simulink model "ScriptDemo"  (R2022b)
settings: configuration reference "TmVcThermal_Configuration_sub" (kept outside this file)
undefined symbols (not defined in the file or in its folder): aaaa, bbbb, cTmComprCtrl_D_u8HvacFlowTable_db, cTmComprCtrl_D_u8HvacFlowTable_sw, cTmComprCtrl_n_i16ChillCmpIMax, cTmComprCtrl_n_i16ChillCmpIMin, cTmComprCtrl_n_i16ChillCmpIMin666, cTmComprCtrl_n_i16ChillCmpPMax, cTmComprCtrl_n_i16ChillCmpPMin, cTmComprCtrl_n_i16CmpChillCoolRpmKiMax, cTmComprCtrl_n_i16CmpChillCoolRpmKiMin, cTmComprCtrl_n_i16CmpChillCoolRpmKpMax, cTmComprCtrl_n_i16CmpChillCoolRpmKpMin, cTmComprCtrl_n_i16CmpCoolRpmKiMax, cTmComprCtrl_n_i16CmpCoolRpmKiMin, cTmComprCtrl_n_i16CmpCoolRpmKpMax, cTmComprCtrl_n_i16CmpCoolRpmKpMin, cTmComprCtrl_n_i16SM4CmpHeatKiMax, cTmComprCtrl_n_i16SM4CmpHeatKiMin, cTmComprCtrl_n_i16SM4CmpHeatKpMax, cTmComprCtrl_n_i16SM4CmpHeatKpMin, cTmComprCtrl_n_i16SM5CmpHeatKiMax, cTmComprCtrl_n_i16SM5CmpHeatKiMin, cTmComprCtrl_n_i16SM5CmpHeatKpMax, cTmComprCtrl_n_i16SM5CmpHeatKpMin, cTmComprCtrl_n_i16SM6CmpHeatKiMax, cTmComprCtrl_n_i16SM6CmpHeatKiMin, cTmComprCtrl_n_i16SM6CmpHeatKpMax, cTmComprCtrl_n_i16SM6CmpHeatKpMin, cTmComprCtrl_n_u16CmpMaxSpdFanFltLimt, cTmComprCtrl_n_u16CmpMaxSpdLoSidePFltLimt, cTmComprCtrl_n_u16CmpMaxSpdSensorFltLimt, cTmComprCtrl_n_u16CompMinRpm, cTmComprCtrl_n_u16CompRpmIncThres, cTmComprCtrl_t_u16BattCooltFFPeriod, cTmComprCtrl_t_u16BattCooltPIPeriod, cTmComprCtrl_t_u16CmpCoolFFPeriod, cTmComprCtrl_t_u16CmpCoolPIPeriod, cTmComprCtrl_t_u16CoolCmpChillFFPeriod, cTmComprCtrl_t_u16CoolCmpChillPIPeriod, cTmComprCtrl_t_u16SM4CmpHeatFFPeriod, cTmComprCtrl_t_u16SM4CmpHeatPIPeriod, cTmComprCtrl_t_u16SM5CmpHeatFFPeriod, cTmComprCtrl_t_u16SM5CmpHeatPIPeriod, cTmComprCtrl_t_u16SM6CmpHeatFFPeriod, cTmComprCtrl_t_u16SM6CmpHeatPIPeriod, cTmComprCtrl_Te_EvapClearInteg, cTmComprCtrl_Te_i16HpReqTempSaturoffset, cTmComprCtrl_Te_i16SatLpReplaceDiff, cTmComprCtrl_Te_i16SM3BatDiffStartEvapDecOffset, cTmComprCtrl_Te_i16SM3EvapLo, cTmComprCtrl_Te_i16SM3TBatDiffEntEvapDecOffset, cTmComprCtrl_Te_i16SM3TBatDiffEntEvapDecOffsetQuit, cTmComprCtrl_Te_s32ErrCmpChillPIContinueCoolH, cTmComprCtrl_Te_s32ErrCmpChillPIContinueCoolL, cTmComprCtrl_Te_s32ErrCmpPIContinueChillH, cTmComprCtrl_Te_s32ErrCmpPIContinueChillL, cTmComprCtrl_Te_s32ErrCmpPIContinueCoolH, cTmComprCtrl_Te_s32ErrCmpPIContinueCoolL, cTmComprCtrl_Te_s32ErrCmpPIContinueHeatH ... (+398)
libraries: simulink x846, PCMULib x711, simulink_need_slupdate x4
(part 23 of 49)

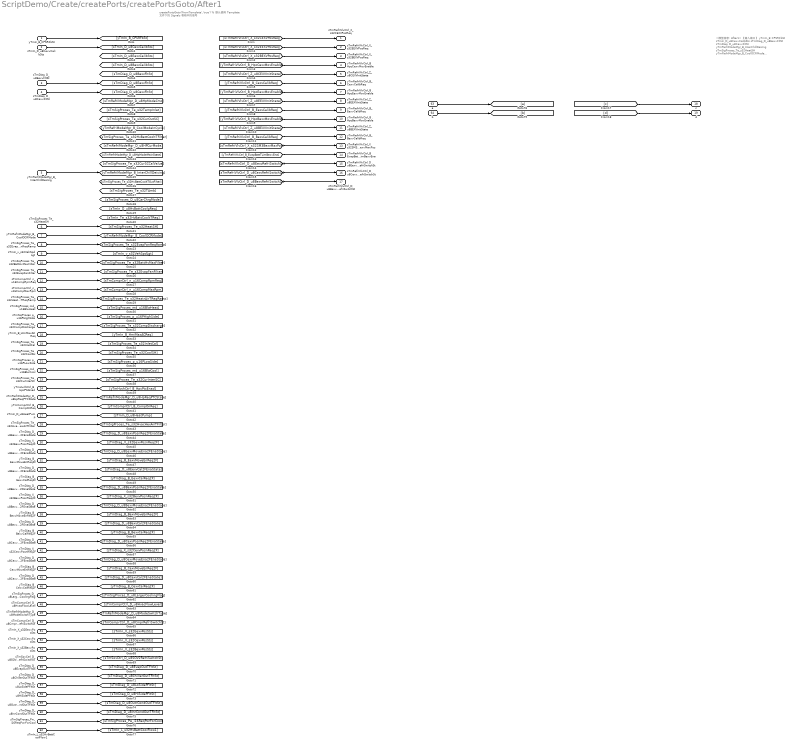
== system ScriptDemo/Create/createPorts/createPortsGoto/After1 ==
  note: createPortsGoto('fromTemplate','true')
      | % 默认使用 Template 文件下的 Signals 表格中的信号
  note: <模型信息: After1>
      |
      |
      | 【输入端口】
      | yTmIn_B_CPSRFbSt
      | sTmIn_D_u8CexvCalibSts
      | sTmDiag_D_u8EexvFltSt
      | sTmDiag_D_u8CexvFltSt
      | yTmRefriModeMgr_B_InterChillDeicing
      | sTmSigProces_Te_s32HeatSH
      | yTmRefriModeMgr_B_CoolOCRMode
      | sTmSigProces_Te_s32EvapFanReqRamp
      | sTmIn_v_s32VehSpdLgt
      | sTmSigProces_Te_s32BattHvMaxFilter
      | sTmSigProces_Te_s32EvapFanFilter
      | sTmComprCtrl_n_u16CompRpmReq
      | sTmComprCtrl_n_u16CompMaxRpm
      | sTmSigProces_Te_s32HeatrAirTReqRamp
      | sTmSigProces_md_u16BlwHeat
      | sTmSigProces_p_u16PHighSide
      | sTmSigProces_Te_s32CompDischarge
      | yTmIn_B_HmiMaxACReq
      | sTmSigProces_Te_s32InletCal
      | sTmSigProces_Te_s32CoolSH
      | sTmSigProces_p_u16PLowSide
      | sTmSigProces_md_u16BlwCool
      | sTmSigProces_Te_s32CurInterSC
      | yTmHvchCtrl_B_HpcPtcEnad
      | sTmRefriModeMgr_D_u8HpReqPTCState
      | yTmComprCtrl_B_CompOnReq
      | sTmIn_D_u8HeatPump
      | sTmSigProces_Te_s32HvacHexAirTFilter
      | sTmDiag_D_u8EexvPosnReq2FEnaState
      | sTmDiag_X_s32EexvPosnReq2F
      | sTmDiag_D_u8EexvMoveEna2FEnaState
      | yTmDiag_B_EexvMoveEnReq2F
      | sTmDiag_D_u8EexvCal2FEnaState
      | yTmDiag_B_EexvCalReq2F
      | sTmDiag_D_u8BexvPosnReq2FEnaState
      | sTmDiag_X_s32BexvPosnReq2F
      | sTmDiag_D_u8BexvMoveEna2FEnaState
      | yTmDiag_B_BexvMoveEnReq2F
      | sTmDiag_D_u8BexvCal2FEnaState
      | yTmDiag_B_BexvCalReq2F
      | sTmDiag_D_u8CexvPosnReq2FEnaState
      | sTmDiag_X_s32CexvPosnReq2F
      | sTmDiag_D_u8CexvMoveEna2FEnaState
      | yTmDiag_B_CexvMoveEnReq2F
      | sTmDiag_D_u8CexvCal2FEnaState
      | yTmDiag_B_CexvCalReq2F
      | sTmSigProces_D_u8LargerCoolingFlag
      | sTmComprCtrl_D_u8HvacFlowLevel
      | sTmRefriModeMgr_D_u8ModeSwitchType
      | sTmComprCtrl_D_u8CmprRefriSwitchSt
      | sTmIn_X_s32EexvPosSts
      | sTmIn_X_s32CexvPosSts
      | sTmIn_X_s32BexvPosSts
      | sTmSovCtrl_D_u8SOV2RefriSwitchSt
      | sTmDiag_D_u8EvapOutTFltSt
      | sTmDiag_D_u8ChillerOutTFltSt
      | sTmDiag_D_u8LoSidePFltSt
      | sTmDiag_D_u8HiSidePFltSt
      | sTmDiag_D_u8OutrCondOutTFltSt
      | sTmDiag_D_u8InrCondOutTFltSt
      | sTmSigProces_Pw_i16ReqPwrForCool
      | sTmIn_L_s32HvBattCoolFlow1
      | a
      | b
      |
      | 【输出端口】
      | sTmRefriVlvCtrl_X_s32CEXVPosReq
      | sTmRefriVlvCtrl_X_s32EEXVPosReq
      | sTmRefriVlvCtrl_X_s32BEXVPosReq
      | yTmRefriVlvCtrl_B_HpcCexvMovEnable
      | sTmRefriVlvCtrl_Z_u8CEXVInitState
      | yTmRefriVlvCtrl_B_CexvCalibReq
      | yTmRefriVlvCtrl_B_HpcEexvMovEnable
      | sTmRefriVlvCtrl_Z_u8EEXVInitState
      | yTmRefriVlvCtrl_B_EexvCalibReq
      | yTmRefriVlvCtrl_B_HpcBexvMovEnable
      | sTmRefriVlvCtrl_Z_u8BEXVInitState
      | yTmRefriVlvCtrl_B_BexvCalibReq
      | sTmRefriVlvCtrl_X_s32SM3BexvMaxPos
      | yTmRefriVlvCtrl_B_EvapBattTLimBexvEna
      | sTmRefriVlvCtrl_D_u8EexvRefriSwitchSt
      | sTmRefriVlvCtrl_D_u8CexvRefriSwitchSt
      | sTmRefriVlvCtrl_D_u8BexvRefriSwitchSt
      | c
      | d
      |
      | 【标定量】
      | 无标定量
      |
      | 创建时间: 2025-05-07 16:48:56
  yTmIn_B_CPSRFbSt : Inport  OutDataTypeStr=boolean
  sTmIn_D_u8CexvCalibSts : Inport  Port=2  OutDataTypeStr=uint8
  sTmDiag_D_u8EexvFltSt : Inport  Port=3  OutDataTypeStr=uint8
  sTmDiag_D_u8CexvFltSt : Inport  Port=4  OutDataTypeStr=uint8
  yTmRefriModeMgr_B_InterChillDeicing : Inport  Port=5  OutDataTypeStr=boolean
  sTmSigProces_Te_s32HeatSH : Inport  Port=6  OutDataTypeStr=single
  yTmRefriModeMgr_B_CoolOCRMode : Inport  Port=7  OutDataTypeStr=boolean
  sTmSigProces_Te_s32EvapFanReqRamp : Inport  Port=8  OutDataTypeStr=single
  sTmIn_v_s32VehSpdLgt : Inport  Port=9  OutDataTypeStr=single
  sTmSigProces_Te_s32BattHvMaxFilter : Inport  Port=10  OutDataTypeStr=single
  sTmSigProces_Te_s32EvapFanFilter : Inport  Port=11  OutDataTypeStr=single
  sTmComprCtrl_n_u16CompRpmReq : Inport  Port=12  OutDataTypeStr=uint16
  sTmComprCtrl_n_u16CompMaxRpm : Inport  Port=13  OutDataTypeStr=uint16
  sTmSigProces_Te_s32HeatrAirTReqRamp : Inport  Port=14  OutDataTypeStr=single
  sTmSigProces_md_u16BlwHeat : Inport  Port=15  OutDataTypeStr=uint16
  sTmSigProces_p_u16PHighSide : Inport  Port=16  OutDataTypeStr=uint16
  sTmSigProces_Te_s32CompDischarge : Inport  Port=17  OutDataTypeStr=single
  yTmIn_B_HmiMaxACReq : Inport  Port=18  OutDataTypeStr=boolean
  sTmSigProces_Te_s32InletCal : Inport  Port=19  OutDataTypeStr=single
  sTmSigProces_Te_s32CoolSH : Inport  Port=20  OutDataTypeStr=single
  sTmSigProces_p_u16PLowSide : Inport  Port=21  OutDataTypeStr=uint16
  sTmSigProces_md_u16BlwCool : Inport  Port=22  OutDataTypeStr=uint16
  sTmSigProces_Te_s32CurInterSC : Inport  Port=23  OutDataTypeStr=single
  yTmHvchCtrl_B_HpcPtcEnad : Inport  Port=24  OutDataTypeStr=boolean
  sTmRefriModeMgr_D_u8HpReqPTCState : Inport  Port=25  OutDataTypeStr=uint8
  yTmComprCtrl_B_CompOnReq : Inport  Port=26  OutDataTypeStr=boolean
  sTmIn_D_u8HeatPump : Inport  Port=27  OutDataTypeStr=uint8
  sTmSigProces_Te_s32HvacHexAirTFilter : Inport  Port=28  OutDataTypeStr=single
  sTmDiag_D_u8EexvPosnReq2FEnaState : Inport  Port=29  OutDataTypeStr=uint8
  sTmDiag_X_s32EexvPosnReq2F : Inport  Port=30  OutDataTypeStr=single
  sTmDiag_D_u8EexvMoveEna2FEnaState : Inport  Port=31  OutDataTypeStr=uint8
  yTmDiag_B_EexvMoveEnReq2F : Inport  Port=32  OutDataTypeStr=boolean
  sTmDiag_D_u8EexvCal2FEnaState : Inport  Port=33  OutDataTypeStr=uint8
  yTmDiag_B_EexvCalReq2F : Inport  Port=34  OutDataTypeStr=boolean
  sTmDiag_D_u8BexvPosnReq2FEnaState : Inport  Port=35  OutDataTypeStr=uint8
  sTmDiag_X_s32BexvPosnReq2F : Inport  Port=36  OutDataTypeStr=single
  sTmDiag_D_u8BexvMoveEna2FEnaState : Inport  Port=37  OutDataTypeStr=uint8
  yTmDiag_B_BexvMoveEnReq2F : Inport  Port=38  OutDataTypeStr=boolean
  sTmDiag_D_u8BexvCal2FEnaState : Inport  Port=39  OutDataTypeStr=uint8
  yTmDiag_B_BexvCalReq2F : Inport  Port=40  OutDataTypeStr=boolean
  sTmDiag_D_u8CexvPosnReq2FEnaState : Inport  Port=41  OutDataTypeStr=uint8
  sTmDiag_X_s32CexvPosnReq2F : Inport  Port=42  OutDataTypeStr=single
  sTmDiag_D_u8CexvMoveEna2FEnaState : Inport  Port=43  OutDataTypeStr=uint8
  yTmDiag_B_CexvMoveEnReq2F : Inport  Port=44  OutDataTypeStr=boolean
  sTmDiag_D_u8CexvCal2FEnaState : Inport  Port=45  OutDataTypeStr=uint8
  yTmDiag_B_CexvCalReq2F : Inport  Port=46  OutDataTypeStr=boolean
  sTmSigProces_D_u8LargerCoolingFlag : Inport  Port=47  OutDataTypeStr=uint8
  sTmComprCtrl_D_u8HvacFlowLevel : Inport  Port=48  OutDataTypeStr=uint8
  sTmRefriModeMgr_D_u8ModeSwitchType : Inport  Port=49  OutDataTypeStr=uint8
  sTmComprCtrl_D_u8CmprRefriSwitchSt : Inport  Port=50  OutDataTypeStr=uint8
  sTmIn_X_s32EexvPosSts : Inport  Port=51  OutDataTypeStr=single
  sTmIn_X_s32CexvPosSts : Inport  Port=52  OutDataTypeStr=single
  sTmIn_X_s32BexvPosSts : Inport  Port=53  OutDataTypeStr=single
  sTmSovCtrl_D_u8SOV2RefriSwitchSt : Inport  Port=54  OutDataTypeStr=uint8
  sTmDiag_D_u8EvapOutTFltSt : Inport  Port=55  OutDataTypeStr=uint8
  sTmDiag_D_u8ChillerOutTFltSt : Inport  Port=56  OutDataTypeStr=uint8
  sTmDiag_D_u8LoSidePFltSt : Inport  Port=57  OutDataTypeStr=uint8
  sTmDiag_D_u8HiSidePFltSt : Inport  Port=58  OutDataTypeStr=uint8
  sTmDiag_D_u8OutrCondOutTFltSt : Inport  Port=59  OutDataTypeStr=uint8
  sTmDiag_D_u8InrCondOutTFltSt : Inport  Port=60  OutDataTypeStr=uint8
  sTmSigProces_Pw_i16ReqPwrForCool : Inport  Port=61  OutDataTypeStr=int16
  sTmIn_L_s32HvBattCoolFlow1 : Inport  Port=62  OutDataTypeStr=single
  a : Inport  Port=63
  b : Inport  Port=64
  sTmRefriVlvCtrl_X_s32CEXVPosReq : Outport  OutDataTypeStr=single
  sTmRefriVlvCtrl_X_s32EEXVPosReq : Outport  Port=2  OutDataTypeStr=single
  sTmRefriVlvCtrl_X_s32BEXVPosReq : Outport  Port=3  OutDataTypeStr=single
  yTmRefriVlvCtrl_B_HpcCexvMovEnable : Outport  Port=4  OutDataTypeStr=boolean
  sTmRefriVlvCtrl_Z_u8CEXVInitState : Outport  Port=5  OutDataTypeStr=uint8
  yTmRefriVlvCtrl_B_CexvCalibReq : Outport  Port=6  OutDataTypeStr=boolean
  yTmRefriVlvCtrl_B_HpcEexvMovEnable : Outport  Port=7  OutDataTypeStr=boolean
  sTmRefriVlvCtrl_Z_u8EEXVInitState : Outport  Port=8  OutDataTypeStr=uint8
  yTmRefriVlvCtrl_B_EexvCalibReq : Outport  Port=9  OutDataTypeStr=boolean
  yTmRefriVlvCtrl_B_HpcBexvMovEnable : Outport  Port=10  OutDataTypeStr=boolean
  sTmRefriVlvCtrl_Z_u8BEXVInitState : Outport  Port=11  OutDataTypeStr=uint8
  yTmRefriVlvCtrl_B_BexvCalibReq : Outport  Port=12  OutDataTypeStr=boolean
  sTmRefriVlvCtrl_X_s32SM3BexvMaxPos : Outport  Port=13  OutDataTypeStr=single
  yTmRefriVlvCtrl_B_EvapBattTLimBexvEna : Outport  Port=14  OutDataTypeStr=boolean
  sTmRefriVlvCtrl_D_u8EexvRefriSwitchSt : Outport  Port=15  OutDataTypeStr=uint8
  sTmRefriVlvCtrl_D_u8CexvRefriSwitchSt : Outport  Port=16  OutDataTypeStr=uint8
  sTmRefriVlvCtrl_D_u8BexvRefriSwitchSt : Outport  Port=17  OutDataTypeStr=uint8
  c : Outport  Port=18
  d : Outport  Port=19
  wires:
  yTmIn_B_CPSRFbSt/1 -> [yTmIn_B_CPSRFbSt]
  sTmIn_D_u8CexvCalibSts/1 -> [sTmIn_D_u8CexvCalibSts]
  ? -> [sTmIn_D_u8EexvCalibSts]
  ? -> [sTmIn_D_u8BexvCalibSts]
  ? -> [sTmDiag_D_u8BexvFltSt]
  sTmDiag_D_u8EexvFltSt/1 -> [sTmDiag_D_u8EexvFltSt]
  sTmDiag_D_u8CexvFltSt/1 -> [sTmDiag_D_u8CexvFltSt]
  ? -> [sTmRefriModeMgr_D_u8HpModeCmd]
  ? -> [sTmSigProces_Te_s32TempInlet]
  ? -> [sTmSigProces_Te_s32CurOutSC]
  ? -> [yTmRefriModeMgr_B_CoolModeInCycle]
  ? -> [sTmSigProces_Te_s32HvBattCooltTFilter]
  ? -> [sTmRefriModeMgr_D_u8HPCurMode]
  ? -> [sTmRefriModeMgr_D_u8HpModeMainState]
  ? -> [sTmSigProces_Te_s32CurSCCalValue]
  yTmRefriModeMgr_B_InterChillDeicing/1 -> [yTmRefriModeMgr_B_InterChillDeicing]
  ? -> [sTmSigProces_Te_s32HvBattCooltTOutFilter]
  ? -> [sTmSigProces_Te_s32TAmb]
  ? -> [sTmSigProces_D_u8CarChrgMode]
  ? -> [sTmIn_D_u8HvBattCoolgReq]
  ? -> [sTmIn_Te_s32HvBattCooltTReq]
  sTmSigProces_Te_s32HeatSH/1 -> [sTmSigProces_Te_s32HeatSH]
  yTmRefriModeMgr_B_CoolOCRMode/1 -> [yTmRefriModeMgr_B_CoolOCRMode]
  sTmSigProces_Te_s32EvapFanReqRamp/1 -> [sTmSigProces_Te_s32EvapFanReqRamp]
  sTmIn_v_s32VehSpdLgt/1 -> [sTmIn_v_s32VehSpdLgt]
  sTmSigProces_Te_s32BattHvMaxFilter/1 -> [sTmSigProces_Te_s32BattHvMaxFilter]
  sTmSigProces_Te_s32EvapFanFilter/1 -> [sTmSigProces_Te_s32EvapFanFilter]
  sTmComprCtrl_n_u16CompRpmReq/1 -> [sTmComprCtrl_n_u16CompRpmReq]
  sTmComprCtrl_n_u16CompMaxRpm/1 -> [sTmComprCtrl_n_u16CompMaxRpm]
  sTmSigProces_Te_s32HeatrAirTReqRamp/1 -> [sTmSigProces_Te_s32HeatrAirTReqRamp]
  sTmSigProces_md_u16BlwHeat/1 -> [sTmSigProces_md_u16BlwHeat]
  sTmSigProces_p_u16PHighSide/1 -> [sTmSigProces_p_u16PHighSide]
  sTmSigProces_Te_s32CompDischarge/1 -> [sTmSigProces_Te_s32CompDischarge]
  yTmIn_B_HmiMaxACReq/1 -> [yTmIn_B_HmiMaxACReq]
  sTmSigProces_Te_s32InletCal/1 -> [sTmSigProces_Te_s32InletCal]
  sTmSigProces_Te_s32CoolSH/1 -> [sTmSigProces_Te_s32CoolSH]
  sTmSigProces_p_u16PLowSide/1 -> [sTmSigProces_p_u16PLowSide]
  sTmSigProces_md_u16BlwCool/1 -> [sTmSigProces_md_u16BlwCool]
  sTmSigProces_Te_s32CurInterSC/1 -> [sTmSigProces_Te_s32CurInterSC]
  yTmHvchCtrl_B_HpcPtcEnad/1 -> [yTmHvchCtrl_B_HpcPtcEnad]
  sTmRefriModeMgr_D_u8HpReqPTCState/1 -> [sTmRefriModeMgr_D_u8HpReqPTCState]
  yTmComprCtrl_B_CompOnReq/1 -> [yTmComprCtrl_B_CompOnReq]
  sTmIn_D_u8HeatPump/1 -> [sTmIn_D_u8HeatPump]
  sTmSigProces_Te_s32HvacHexAirTFilter/1 -> [sTmSigProces_Te_s32HvacHexAirTFilter]
  sTmDiag_D_u8EexvPosnReq2FEnaState/1 -> [sTmDiag_D_u8EexvPosnReq2FEnaState]
  sTmDiag_X_s32EexvPosnReq2F/1 -> [sTmDiag_X_s32EexvPosnReq2F]
  sTmDiag_D_u8EexvMoveEna2FEnaState/1 -> [sTmDiag_D_u8EexvMoveEna2FEnaState]
  yTmDiag_B_EexvMoveEnReq2F/1 -> [yTmDiag_B_EexvMoveEnReq2F]
  sTmDiag_D_u8EexvCal2FEnaState/1 -> [sTmDiag_D_u8EexvCal2FEnaState]
  yTmDiag_B_EexvCalReq2F/1 -> [yTmDiag_B_EexvCalReq2F]
  sTmDiag_D_u8BexvPosnReq2FEnaState/1 -> [sTmDiag_D_u8BexvPosnReq2FEnaState]
  sTmDiag_X_s32BexvPosnReq2F/1 -> [sTmDiag_X_s32BexvPosnReq2F]
  sTmDiag_D_u8BexvMoveEna2FEnaState/1 -> [sTmDiag_D_u8BexvMoveEna2FEnaState]
  yTmDiag_B_BexvMoveEnReq2F/1 -> [yTmDiag_B_BexvMoveEnReq2F]
  sTmDiag_D_u8BexvCal2FEnaState/1 -> [sTmDiag_D_u8BexvCal2FEnaState]
  yTmDiag_B_BexvCalReq2F/1 -> [yTmDiag_B_BexvCalReq2F]
  sTmDiag_D_u8CexvPosnReq2FEnaState/1 -> [sTmDiag_D_u8CexvPosnReq2FEnaState]
  sTmDiag_X_s32CexvPosnReq2F/1 -> [sTmDiag_X_s32CexvPosnReq2F]
  sTmDiag_D_u8CexvMoveEna2FEnaState/1 -> [sTmDiag_D_u8CexvMoveEna2FEnaState]
  yTmDiag_B_CexvMoveEnReq2F/1 -> [yTmDiag_B_CexvMoveEnReq2F]
  sTmDiag_D_u8CexvCal2FEnaState/1 -> [sTmDiag_D_u8CexvCal2FEnaState]
  yTmDiag_B_CexvCalReq2F/1 -> [yTmDiag_B_CexvCalReq2F]
  sTmSigProces_D_u8LargerCoolingFlag/1 -> [sTmSigProces_D_u8LargerCoolingFlag]
  sTmComprCtrl_D_u8HvacFlowLevel/1 -> [sTmComprCtrl_D_u8HvacFlowLevel]
  sTmRefriModeMgr_D_u8ModeSwitchType/1 -> [sTmRefriModeMgr_D_u8ModeSwitchType]
  sTmComprCtrl_D_u8CmprRefriSwitchSt/1 -> [sTmComprCtrl_D_u8CmprRefriSwitchSt]
  sTmIn_X_s32EexvPosSts/1 -> [sTmIn_X_s32EexvPosSts]
  sTmIn_X_s32CexvPosSts/1 -> [sTmIn_X_s32CexvPosSts]
  sTmIn_X_s32BexvPosSts/1 -> [sTmIn_X_s32BexvPosSts]
  sTmSovCtrl_D_u8SOV2RefriSwitchSt/1 -> [sTmSovCtrl_D_u8SOV2RefriSwitchSt]
  sTmDiag_D_u8EvapOutTFltSt/1 -> [sTmDiag_D_u8EvapOutTFltSt]
  sTmDiag_D_u8ChillerOutTFltSt/1 -> [sTmDiag_D_u8ChillerOutTFltSt]
  sTmDiag_D_u8LoSidePFltSt/1 -> [sTmDiag_D_u8LoSidePFltSt]
  sTmDiag_D_u8HiSidePFltSt/1 -> [sTmDiag_D_u8HiSidePFltSt]
  sTmDiag_D_u8OutrCondOutTFltSt/1 -> [sTmDiag_D_u8OutrCondOutTFltSt]
  sTmDiag_D_u8InrCondOutTFltSt/1 -> [sTmDiag_D_u8InrCondOutTFltSt]
  sTmSigProces_Pw_i16ReqPwrForCool/1 -> [sTmSigProces_Pw_i16ReqPwrForCool]
  sTmIn_L_s32HvBattCoolFlow1/1 -> [sTmIn_L_s32HvBattCoolFlow1]
  [sTmRefriVlvCtrl_X_s32CEXVPosReq] -> sTmRefriVlvCtrl_X_s32CEXVPosReq/1
  [sTmRefriVlvCtrl_X_s32EEXVPosReq] -> sTmRefriVlvCtrl_X_s32EEXVPosReq/1
  [sTmRefriVlvCtrl_X_s32BEXVPosReq] -> sTmRefriVlvCtrl_X_s32BEXVPosReq/1
  [yTmRefriVlvCtrl_B_HpcCexvMovEnable] -> yTmRefriVlvCtrl_B_HpcCexvMovEnable/1
  [sTmRefriVlvCtrl_Z_u8CEXVInitState] -> sTmRefriVlvCtrl_Z_u8CEXVInitState/1
  [yTmRefriVlvCtrl_B_CexvCalibReq] -> yTmRefriVlvCtrl_B_CexvCalibReq/1
  [yTmRefriVlvCtrl_B_HpcEexvMovEnable] -> yTmRefriVlvCtrl_B_HpcEexvMovEnable/1
  [sTmRefriVlvCtrl_Z_u8EEXVInitState] -> sTmRefriVlvCtrl_Z_u8EEXVInitState/1
  [yTmRefriVlvCtrl_B_EexvCalibReq] -> yTmRefriVlvCtrl_B_EexvCalibReq/1
  [yTmRefriVlvCtrl_B_HpcBexvMovEnable] -> yTmRefriVlvCtrl_B_HpcBexvMovEnable/1
  [sTmRefriVlvCtrl_Z_u8BEXVInitState] -> sTmRefriVlvCtrl_Z_u8BEXVInitState/1
  [yTmRefriVlvCtrl_B_BexvCalibReq] -> yTmRefriVlvCtrl_B_BexvCalibReq/1
  [sTmRefriVlvCtrl_X_s32SM3BexvMaxPos] -> sTmRefriVlvCtrl_X_s32SM3BexvMaxPos/1
  [yTmRefriVlvCtrl_B_EvapBattTLimBexvEna] -> yTmRefriVlvCtrl_B_EvapBattTLimBexvEna/1
  [sTmRefriVlvCtrl_D_u8EexvRefriSwitchSt] -> sTmRefriVlvCtrl_D_u8EexvRefriSwitchSt/1
  [sTmRefriVlvCtrl_D_u8CexvRefriSwitchSt] -> sTmRefriVlvCtrl_D_u8CexvRefriSwitchSt/1
  [sTmRefriVlvCtrl_D_u8BexvRefriSwitchSt] -> sTmRefriVlvCtrl_D_u8BexvRefriSwitchSt/1
  a/1 -> [a]
  b/1 -> [b]
  [c] -> c/1
  [d] -> d/1

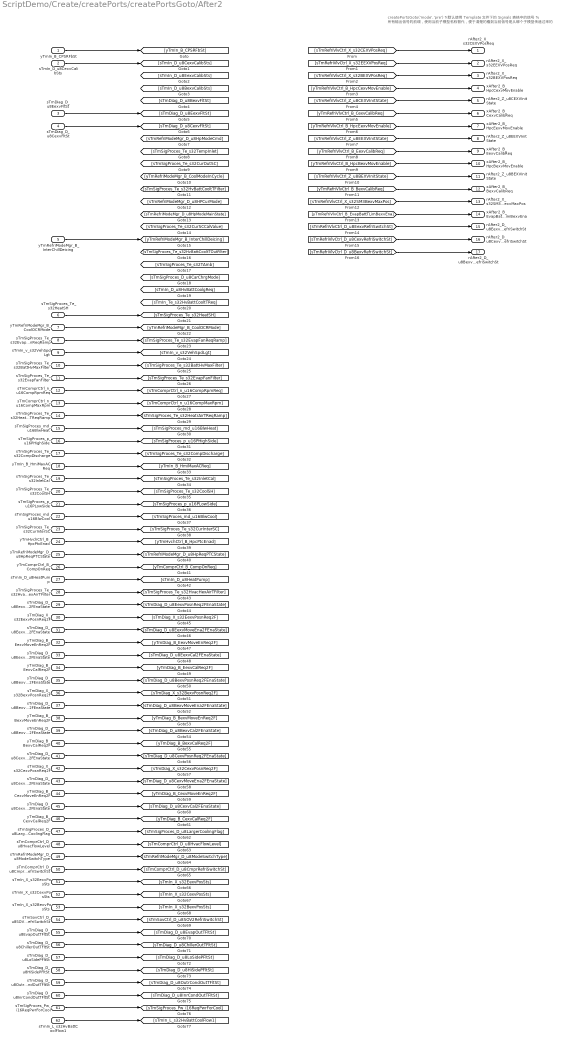
== system ScriptDemo/Create/createPorts/createPortsGoto/After2 ==
  note: createPortsGoto('mode','pre')
      | % 默认使用 Template 文件下的 Signals 表格中的信号
      | % 所有输出信号的前缀，使用当前子模型名称替代，便于清楚的看到当前信号是从哪个子模型传递过来的
  yTmIn_B_CPSRFbSt : Inport  OutDataTypeStr=boolean
  sTmIn_D_u8CexvCalibSts : Inport  Port=2  OutDataTypeStr=uint8
  sTmDiag_D_u8EexvFltSt : Inport  Port=3  OutDataTypeStr=uint8
  sTmDiag_D_u8CexvFltSt : Inport  Port=4  OutDataTypeStr=uint8
  yTmRefriModeMgr_B_InterChillDeicing : Inport  Port=5  OutDataTypeStr=boolean
  sTmSigProces_Te_s32HeatSH : Inport  Port=6  OutDataTypeStr=single
  yTmRefriModeMgr_B_CoolOCRMode : Inport  Port=7  OutDataTypeStr=boolean
  sTmSigProces_Te_s32EvapFanReqRamp : Inport  Port=8  OutDataTypeStr=single
  sTmIn_v_s32VehSpdLgt : Inport  Port=9  OutDataTypeStr=single
  sTmSigProces_Te_s32BattHvMaxFilter : Inport  Port=10  OutDataTypeStr=single
  sTmSigProces_Te_s32EvapFanFilter : Inport  Port=11  OutDataTypeStr=single
  sTmComprCtrl_n_u16CompRpmReq : Inport  Port=12  OutDataTypeStr=uint16
  sTmComprCtrl_n_u16CompMaxRpm : Inport  Port=13  OutDataTypeStr=uint16
  sTmSigProces_Te_s32HeatrAirTReqRamp : Inport  Port=14  OutDataTypeStr=single
  sTmSigProces_md_u16BlwHeat : Inport  Port=15  OutDataTypeStr=uint16
  sTmSigProces_p_u16PHighSide : Inport  Port=16  OutDataTypeStr=uint16
  sTmSigProces_Te_s32CompDischarge : Inport  Port=17  OutDataTypeStr=single
  yTmIn_B_HmiMaxACReq : Inport  Port=18  OutDataTypeStr=boolean
  sTmSigProces_Te_s32InletCal : Inport  Port=19  OutDataTypeStr=single
  sTmSigProces_Te_s32CoolSH : Inport  Port=20  OutDataTypeStr=single
  sTmSigProces_p_u16PLowSide : Inport  Port=21  OutDataTypeStr=uint16
  sTmSigProces_md_u16BlwCool : Inport  Port=22  OutDataTypeStr=uint16
  sTmSigProces_Te_s32CurInterSC : Inport  Port=23  OutDataTypeStr=single
  yTmHvchCtrl_B_HpcPtcEnad : Inport  Port=24  OutDataTypeStr=boolean
  sTmRefriModeMgr_D_u8HpReqPTCState : Inport  Port=25  OutDataTypeStr=uint8
  yTmComprCtrl_B_CompOnReq : Inport  Port=26  OutDataTypeStr=boolean
  sTmIn_D_u8HeatPump : Inport  Port=27  OutDataTypeStr=uint8
  sTmSigProces_Te_s32HvacHexAirTFilter : Inport  Port=28  OutDataTypeStr=single
  sTmDiag_D_u8EexvPosnReq2FEnaState : Inport  Port=29  OutDataTypeStr=uint8
  sTmDiag_X_s32EexvPosnReq2F : Inport  Port=30  OutDataTypeStr=single
  sTmDiag_D_u8EexvMoveEna2FEnaState : Inport  Port=31  OutDataTypeStr=uint8
  yTmDiag_B_EexvMoveEnReq2F : Inport  Port=32  OutDataTypeStr=boolean
  sTmDiag_D_u8EexvCal2FEnaState : Inport  Port=33  OutDataTypeStr=uint8
  yTmDiag_B_EexvCalReq2F : Inport  Port=34  OutDataTypeStr=boolean
  sTmDiag_D_u8BexvPosnReq2FEnaState : Inport  Port=35  OutDataTypeStr=uint8
  sTmDiag_X_s32BexvPosnReq2F : Inport  Port=36  OutDataTypeStr=single
  sTmDiag_D_u8BexvMoveEna2FEnaState : Inport  Port=37  OutDataTypeStr=uint8
  yTmDiag_B_BexvMoveEnReq2F : Inport  Port=38  OutDataTypeStr=boolean
  sTmDiag_D_u8BexvCal2FEnaState : Inport  Port=39  OutDataTypeStr=uint8
  yTmDiag_B_BexvCalReq2F : Inport  Port=40  OutDataTypeStr=boolean
  sTmDiag_D_u8CexvPosnReq2FEnaState : Inport  Port=41  OutDataTypeStr=uint8
  sTmDiag_X_s32CexvPosnReq2F : Inport  Port=42  OutDataTypeStr=single
  sTmDiag_D_u8CexvMoveEna2FEnaState : Inport  Port=43  OutDataTypeStr=uint8
  yTmDiag_B_CexvMoveEnReq2F : Inport  Port=44  OutDataTypeStr=boolean
  sTmDiag_D_u8CexvCal2FEnaState : Inport  Port=45  OutDataTypeStr=uint8
  yTmDiag_B_CexvCalReq2F : Inport  Port=46  OutDataTypeStr=boolean
  sTmSigProces_D_u8LargerCoolingFlag : Inport  Port=47  OutDataTypeStr=uint8
  sTmComprCtrl_D_u8HvacFlowLevel : Inport  Port=48  OutDataTypeStr=uint8
  sTmRefriModeMgr_D_u8ModeSwitchType : Inport  Port=49  OutDataTypeStr=uint8
  sTmComprCtrl_D_u8CmprRefriSwitchSt : Inport  Port=50  OutDataTypeStr=uint8
  sTmIn_X_s32EexvPosSts : Inport  Port=51  OutDataTypeStr=single
  sTmIn_X_s32CexvPosSts : Inport  Port=52  OutDataTypeStr=single
  sTmIn_X_s32BexvPosSts : Inport  Port=53  OutDataTypeStr=single
  sTmSovCtrl_D_u8SOV2RefriSwitchSt : Inport  Port=54  OutDataTypeStr=uint8
  sTmDiag_D_u8EvapOutTFltSt : Inport  Port=55  OutDataTypeStr=uint8
  sTmDiag_D_u8ChillerOutTFltSt : Inport  Port=56  OutDataTypeStr=uint8
  sTmDiag_D_u8LoSidePFltSt : Inport  Port=57  OutDataTypeStr=uint8
  sTmDiag_D_u8HiSidePFltSt : Inport  Port=58  OutDataTypeStr=uint8
  sTmDiag_D_u8OutrCondOutTFltSt : Inport  Port=59  OutDataTypeStr=uint8
  sTmDiag_D_u8InrCondOutTFltSt : Inport  Port=60  OutDataTypeStr=uint8
  sTmSigProces_Pw_i16ReqPwrForCool : Inport  Port=61  OutDataTypeStr=int16
  sTmIn_L_s32HvBattCoolFlow1 : Inport  Port=62  OutDataTypeStr=single
  rAfter2_X_s32CEXVPosReq : Outport  OutDataTypeStr=single
  rAfter2_X_s32EEXVPosReq : Outport  Port=2  OutDataTypeStr=single
  rAfter2_X_s32BEXVPosReq : Outport  Port=3  OutDataTypeStr=single
  xAfter2_B_HpcCexvMovEnable : Outport  Port=4  OutDataTypeStr=boolean
  rAfter2_Z_u8CEXVInitState : Outport  Port=5  OutDataTypeStr=uint8
  xAfter2_B_CexvCalibReq : Outport  Port=6  OutDataTypeStr=boolean
  xAfter2_B_HpcEexvMovEnable : Outport  Port=7  OutDataTypeStr=boolean
  rAfter2_Z_u8EEXVInitState : Outport  Port=8  OutDataTypeStr=uint8
  xAfter2_B_EexvCalibReq : Outport  Port=9  OutDataTypeStr=boolean
  xAfter2_B_HpcBexvMovEnable : Outport  Port=10  OutDataTypeStr=boolean
  rAfter2_Z_u8BEXVInitState : Outport  Port=11  OutDataTypeStr=uint8
  xAfter2_B_BexvCalibReq : Outport  Port=12  OutDataTypeStr=boolean
  rAfter2_X_s32SM3BexvMaxPos : Outport  Port=13  OutDataTypeStr=single
  xAfter2_B_EvapBattTLimBexvEna : Outport  Port=14  OutDataTypeStr=boolean
  rAfter2_D_u8EexvRefriSwitchSt : Outport  Port=15  OutDataTypeStr=uint8
  rAfter2_D_u8CexvRefriSwitchSt : Outport  Port=16  OutDataTypeStr=uint8
  rAfter2_D_u8BexvRefriSwitchSt : Outport  Port=17  OutDataTypeStr=uint8
  wires:
  yTmIn_B_CPSRFbSt/1 -> [yTmIn_B_CPSRFbSt]
  sTmIn_D_u8CexvCalibSts/1 -> [sTmIn_D_u8CexvCalibSts]
  ? -> [sTmIn_D_u8EexvCalibSts]
  ? -> [sTmIn_D_u8BexvCalibSts]
  ? -> [sTmDiag_D_u8BexvFltSt]
  sTmDiag_D_u8EexvFltSt/1 -> [sTmDiag_D_u8EexvFltSt]
  sTmDiag_D_u8CexvFltSt/1 -> [sTmDiag_D_u8CexvFltSt]
  ? -> [sTmRefriModeMgr_D_u8HpModeCmd]
  ? -> [sTmSigProces_Te_s32TempInlet]
  ? -> [sTmSigProces_Te_s32CurOutSC]
  ? -> [yTmRefriModeMgr_B_CoolModeInCycle]
  ? -> [sTmSigProces_Te_s32HvBattCooltTFilter]
  ? -> [sTmRefriModeMgr_D_u8HPCurMode]
  ? -> [sTmRefriModeMgr_D_u8HpModeMainState]
  ? -> [sTmSigProces_Te_s32CurSCCalValue]
  yTmRefriModeMgr_B_InterChillDeicing/1 -> [yTmRefriModeMgr_B_InterChillDeicing]
  ? -> [sTmSigProces_Te_s32HvBattCooltTOutFilter]
  ? -> [sTmSigProces_Te_s32TAmb]
  ? -> [sTmSigProces_D_u8CarChrgMode]
  ? -> [sTmIn_D_u8HvBattCoolgReq]
  ? -> [sTmIn_Te_s32HvBattCooltTReq]
  sTmSigProces_Te_s32HeatSH/1 -> [sTmSigProces_Te_s32HeatSH]
  yTmRefriModeMgr_B_CoolOCRMode/1 -> [yTmRefriModeMgr_B_CoolOCRMode]
  sTmSigProces_Te_s32EvapFanReqRamp/1 -> [sTmSigProces_Te_s32EvapFanReqRamp]
  sTmIn_v_s32VehSpdLgt/1 -> [sTmIn_v_s32VehSpdLgt]
  sTmSigProces_Te_s32BattHvMaxFilter/1 -> [sTmSigProces_Te_s32BattHvMaxFilter]
  sTmSigProces_Te_s32EvapFanFilter/1 -> [sTmSigProces_Te_s32EvapFanFilter]
  sTmComprCtrl_n_u16CompRpmReq/1 -> [sTmComprCtrl_n_u16CompRpmReq]
  sTmComprCtrl_n_u16CompMaxRpm/1 -> [sTmComprCtrl_n_u16CompMaxRpm]
  sTmSigProces_Te_s32HeatrAirTReqRamp/1 -> [sTmSigProces_Te_s32HeatrAirTReqRamp]
  sTmSigProces_md_u16BlwHeat/1 -> [sTmSigProces_md_u16BlwHeat]
  sTmSigProces_p_u16PHighSide/1 -> [sTmSigProces_p_u16PHighSide]
  sTmSigProces_Te_s32CompDischarge/1 -> [sTmSigProces_Te_s32CompDischarge]
  yTmIn_B_HmiMaxACReq/1 -> [yTmIn_B_HmiMaxACReq]
  sTmSigProces_Te_s32InletCal/1 -> [sTmSigProces_Te_s32InletCal]
  sTmSigProces_Te_s32CoolSH/1 -> [sTmSigProces_Te_s32CoolSH]
  sTmSigProces_p_u16PLowSide/1 -> [sTmSigProces_p_u16PLowSide]
  sTmSigProces_md_u16BlwCool/1 -> [sTmSigProces_md_u16BlwCool]
  sTmSigProces_Te_s32CurInterSC/1 -> [sTmSigProces_Te_s32CurInterSC]
  yTmHvchCtrl_B_HpcPtcEnad/1 -> [yTmHvchCtrl_B_HpcPtcEnad]
  sTmRefriModeMgr_D_u8HpReqPTCState/1 -> [sTmRefriModeMgr_D_u8HpReqPTCState]
  yTmComprCtrl_B_CompOnReq/1 -> [yTmComprCtrl_B_CompOnReq]
  sTmIn_D_u8HeatPump/1 -> [sTmIn_D_u8HeatPump]
  sTmSigProces_Te_s32HvacHexAirTFilter/1 -> [sTmSigProces_Te_s32HvacHexAirTFilter]
  sTmDiag_D_u8EexvPosnReq2FEnaState/1 -> [sTmDiag_D_u8EexvPosnReq2FEnaState]
  sTmDiag_X_s32EexvPosnReq2F/1 -> [sTmDiag_X_s32EexvPosnReq2F]
  sTmDiag_D_u8EexvMoveEna2FEnaState/1 -> [sTmDiag_D_u8EexvMoveEna2FEnaState]
  yTmDiag_B_EexvMoveEnReq2F/1 -> [yTmDiag_B_EexvMoveEnReq2F]
  sTmDiag_D_u8EexvCal2FEnaState/1 -> [sTmDiag_D_u8EexvCal2FEnaState]
  yTmDiag_B_EexvCalReq2F/1 -> [yTmDiag_B_EexvCalReq2F]
  sTmDiag_D_u8BexvPosnReq2FEnaState/1 -> [sTmDiag_D_u8BexvPosnReq2FEnaState]
  sTmDiag_X_s32BexvPosnReq2F/1 -> [sTmDiag_X_s32BexvPosnReq2F]
  sTmDiag_D_u8BexvMoveEna2FEnaState/1 -> [sTmDiag_D_u8BexvMoveEna2FEnaState]
  yTmDiag_B_BexvMoveEnReq2F/1 -> [yTmDiag_B_BexvMoveEnReq2F]
  sTmDiag_D_u8BexvCal2FEnaState/1 -> [sTmDiag_D_u8BexvCal2FEnaState]
  yTmDiag_B_BexvCalReq2F/1 -> [yTmDiag_B_BexvCalReq2F]
  sTmDiag_D_u8CexvPosnReq2FEnaState/1 -> [sTmDiag_D_u8CexvPosnReq2FEnaState]
  sTmDiag_X_s32CexvPosnReq2F/1 -> [sTmDiag_X_s32CexvPosnReq2F]
  sTmDiag_D_u8CexvMoveEna2FEnaState/1 -> [sTmDiag_D_u8CexvMoveEna2FEnaState]
  yTmDiag_B_CexvMoveEnReq2F/1 -> [yTmDiag_B_CexvMoveEnReq2F]
  sTmDiag_D_u8CexvCal2FEnaState/1 -> [sTmDiag_D_u8CexvCal2FEnaState]
  yTmDiag_B_CexvCalReq2F/1 -> [yTmDiag_B_CexvCalReq2F]
  sTmSigProces_D_u8LargerCoolingFlag/1 -> [sTmSigProces_D_u8LargerCoolingFlag]
  sTmComprCtrl_D_u8HvacFlowLevel/1 -> [sTmComprCtrl_D_u8HvacFlowLevel]
  sTmRefriModeMgr_D_u8ModeSwitchType/1 -> [sTmRefriModeMgr_D_u8ModeSwitchType]
  sTmComprCtrl_D_u8CmprRefriSwitchSt/1 -> [sTmComprCtrl_D_u8CmprRefriSwitchSt]
  sTmIn_X_s32EexvPosSts/1 -> [sTmIn_X_s32EexvPosSts]
  sTmIn_X_s32CexvPosSts/1 -> [sTmIn_X_s32CexvPosSts]
  sTmIn_X_s32BexvPosSts/1 -> [sTmIn_X_s32BexvPosSts]
  sTmSovCtrl_D_u8SOV2RefriSwitchSt/1 -> [sTmSovCtrl_D_u8SOV2RefriSwitchSt]
  sTmDiag_D_u8EvapOutTFltSt/1 -> [sTmDiag_D_u8EvapOutTFltSt]
  sTmDiag_D_u8ChillerOutTFltSt/1 -> [sTmDiag_D_u8ChillerOutTFltSt]
  sTmDiag_D_u8LoSidePFltSt/1 -> [sTmDiag_D_u8LoSidePFltSt]
  sTmDiag_D_u8HiSidePFltSt/1 -> [sTmDiag_D_u8HiSidePFltSt]
  sTmDiag_D_u8OutrCondOutTFltSt/1 -> [sTmDiag_D_u8OutrCondOutTFltSt]
  sTmDiag_D_u8InrCondOutTFltSt/1 -> [sTmDiag_D_u8InrCondOutTFltSt]
  sTmSigProces_Pw_i16ReqPwrForCool/1 -> [sTmSigProces_Pw_i16ReqPwrForCool]
  sTmIn_L_s32HvBattCoolFlow1/1 -> [sTmIn_L_s32HvBattCoolFlow1]
  [sTmRefriVlvCtrl_X_s32CEXVPosReq] -> rAfter2_X_s32CEXVPosReq/1
  [sTmRefriVlvCtrl_X_s32EEXVPosReq] -> rAfter2_X_s32EEXVPosReq/1
  [sTmRefriVlvCtrl_X_s32BEXVPosReq] -> rAfter2_X_s32BEXVPosReq/1
  [yTmRefriVlvCtrl_B_HpcCexvMovEnable] -> xAfter2_B_HpcCexvMovEnable/1
  [sTmRefriVlvCtrl_Z_u8CEXVInitState] -> rAfter2_Z_u8CEXVInitState/1
  [yTmRefriVlvCtrl_B_CexvCalibReq] -> xAfter2_B_CexvCalibReq/1
  [yTmRefriVlvCtrl_B_HpcEexvMovEnable] -> xAfter2_B_HpcEexvMovEnable/1
  [sTmRefriVlvCtrl_Z_u8EEXVInitState] -> rAfter2_Z_u8EEXVInitState/1
  [yTmRefriVlvCtrl_B_EexvCalibReq] -> xAfter2_B_EexvCalibReq/1
  [yTmRefriVlvCtrl_B_HpcBexvMovEnable] -> xAfter2_B_HpcBexvMovEnable/1
  [sTmRefriVlvCtrl_Z_u8BEXVInitState] -> rAfter2_Z_u8BEXVInitState/1
  [yTmRefriVlvCtrl_B_BexvCalibReq] -> xAfter2_B_BexvCalibReq/1
  [sTmRefriVlvCtrl_X_s32SM3BexvMaxPos] -> rAfter2_X_s32SM3BexvMaxPos/1
  [yTmRefriVlvCtrl_B_EvapBattTLimBexvEna] -> xAfter2_B_EvapBattTLimBexvEna/1
  [sTmRefriVlvCtrl_D_u8EexvRefriSwitchSt] -> rAfter2_D_u8EexvRefriSwitchSt/1
  [sTmRefriVlvCtrl_D_u8CexvRefriSwitchSt] -> rAfter2_D_u8CexvRefriSwitchSt/1
  [sTmRefriVlvCtrl_D_u8BexvRefriSwitchSt] -> rAfter2_D_u8BexvRefriSwitchSt/1

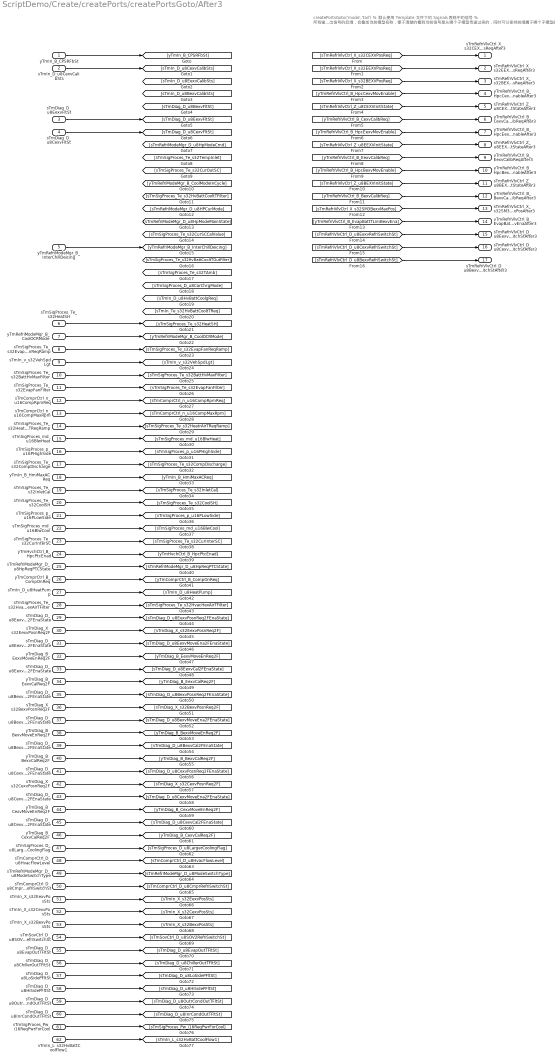
== system ScriptDemo/Create/createPorts/createPortsGoto/After3 ==
  note: createPortsGoto('mode','tail')
      | % 默认使用 Template 文件下的 Signals 表格中的信号
      | % 所有输出信号的后缀，会叠加当前模型名称，便于清楚的看到当前信号是从哪个子模型传递过来的，同时可以保持前缀属于哪个子模型的
  yTmIn_B_CPSRFbSt : Inport  OutDataTypeStr=boolean
  sTmIn_D_u8CexvCalibSts : Inport  Port=2  OutDataTypeStr=uint8
  sTmDiag_D_u8EexvFltSt : Inport  Port=3  OutDataTypeStr=uint8
  sTmDiag_D_u8CexvFltSt : Inport  Port=4  OutDataTypeStr=uint8
  yTmRefriModeMgr_B_InterChillDeicing : Inport  Port=5  OutDataTypeStr=boolean
  sTmSigProces_Te_s32HeatSH : Inport  Port=6  OutDataTypeStr=single
  yTmRefriModeMgr_B_CoolOCRMode : Inport  Port=7  OutDataTypeStr=boolean
  sTmSigProces_Te_s32EvapFanReqRamp : Inport  Port=8  OutDataTypeStr=single
  sTmIn_v_s32VehSpdLgt : Inport  Port=9  OutDataTypeStr=single
  sTmSigProces_Te_s32BattHvMaxFilter : Inport  Port=10  OutDataTypeStr=single
  sTmSigProces_Te_s32EvapFanFilter : Inport  Port=11  OutDataTypeStr=single
  sTmComprCtrl_n_u16CompRpmReq : Inport  Port=12  OutDataTypeStr=uint16
  sTmComprCtrl_n_u16CompMaxRpm : Inport  Port=13  OutDataTypeStr=uint16
  sTmSigProces_Te_s32HeatrAirTReqRamp : Inport  Port=14  OutDataTypeStr=single
  sTmSigProces_md_u16BlwHeat : Inport  Port=15  OutDataTypeStr=uint16
  sTmSigProces_p_u16PHighSide : Inport  Port=16  OutDataTypeStr=uint16
  sTmSigProces_Te_s32CompDischarge : Inport  Port=17  OutDataTypeStr=single
  yTmIn_B_HmiMaxACReq : Inport  Port=18  OutDataTypeStr=boolean
  sTmSigProces_Te_s32InletCal : Inport  Port=19  OutDataTypeStr=single
  sTmSigProces_Te_s32CoolSH : Inport  Port=20  OutDataTypeStr=single
  sTmSigProces_p_u16PLowSide : Inport  Port=21  OutDataTypeStr=uint16
  sTmSigProces_md_u16BlwCool : Inport  Port=22  OutDataTypeStr=uint16
  sTmSigProces_Te_s32CurInterSC : Inport  Port=23  OutDataTypeStr=single
  yTmHvchCtrl_B_HpcPtcEnad : Inport  Port=24  OutDataTypeStr=boolean
  sTmRefriModeMgr_D_u8HpReqPTCState : Inport  Port=25  OutDataTypeStr=uint8
  yTmComprCtrl_B_CompOnReq : Inport  Port=26  OutDataTypeStr=boolean
  sTmIn_D_u8HeatPump : Inport  Port=27  OutDataTypeStr=uint8
  sTmSigProces_Te_s32HvacHexAirTFilter : Inport  Port=28  OutDataTypeStr=single
  sTmDiag_D_u8EexvPosnReq2FEnaState : Inport  Port=29  OutDataTypeStr=uint8
  sTmDiag_X_s32EexvPosnReq2F : Inport  Port=30  OutDataTypeStr=single
  sTmDiag_D_u8EexvMoveEna2FEnaState : Inport  Port=31  OutDataTypeStr=uint8
  yTmDiag_B_EexvMoveEnReq2F : Inport  Port=32  OutDataTypeStr=boolean
  sTmDiag_D_u8EexvCal2FEnaState : Inport  Port=33  OutDataTypeStr=uint8
  yTmDiag_B_EexvCalReq2F : Inport  Port=34  OutDataTypeStr=boolean
  sTmDiag_D_u8BexvPosnReq2FEnaState : Inport  Port=35  OutDataTypeStr=uint8
  sTmDiag_X_s32BexvPosnReq2F : Inport  Port=36  OutDataTypeStr=single
  sTmDiag_D_u8BexvMoveEna2FEnaState : Inport  Port=37  OutDataTypeStr=uint8
  yTmDiag_B_BexvMoveEnReq2F : Inport  Port=38  OutDataTypeStr=boolean
  sTmDiag_D_u8BexvCal2FEnaState : Inport  Port=39  OutDataTypeStr=uint8
  yTmDiag_B_BexvCalReq2F : Inport  Port=40  OutDataTypeStr=boolean
  sTmDiag_D_u8CexvPosnReq2FEnaState : Inport  Port=41  OutDataTypeStr=uint8
  sTmDiag_X_s32CexvPosnReq2F : Inport  Port=42  OutDataTypeStr=single
  sTmDiag_D_u8CexvMoveEna2FEnaState : Inport  Port=43  OutDataTypeStr=uint8
  yTmDiag_B_CexvMoveEnReq2F : Inport  Port=44  OutDataTypeStr=boolean
  sTmDiag_D_u8CexvCal2FEnaState : Inport  Port=45  OutDataTypeStr=uint8
  yTmDiag_B_CexvCalReq2F : Inport  Port=46  OutDataTypeStr=boolean
  sTmSigProces_D_u8LargerCoolingFlag : Inport  Port=47  OutDataTypeStr=uint8
  sTmComprCtrl_D_u8HvacFlowLevel : Inport  Port=48  OutDataTypeStr=uint8
  sTmRefriModeMgr_D_u8ModeSwitchType : Inport  Port=49  OutDataTypeStr=uint8
  sTmComprCtrl_D_u8CmprRefriSwitchSt : Inport  Port=50  OutDataTypeStr=uint8
  sTmIn_X_s32EexvPosSts : Inport  Port=51  OutDataTypeStr=single
  sTmIn_X_s32CexvPosSts : Inport  Port=52  OutDataTypeStr=single
  sTmIn_X_s32BexvPosSts : Inport  Port=53  OutDataTypeStr=single
  sTmSovCtrl_D_u8SOV2RefriSwitchSt : Inport  Port=54  OutDataTypeStr=uint8
  sTmDiag_D_u8EvapOutTFltSt : Inport  Port=55  OutDataTypeStr=uint8
  sTmDiag_D_u8ChillerOutTFltSt : Inport  Port=56  OutDataTypeStr=uint8
  sTmDiag_D_u8LoSidePFltSt : Inport  Port=57  OutDataTypeStr=uint8
  sTmDiag_D_u8HiSidePFltSt : Inport  Port=58  OutDataTypeStr=uint8
  sTmDiag_D_u8OutrCondOutTFltSt : Inport  Port=59  OutDataTypeStr=uint8
  sTmDiag_D_u8InrCondOutTFltSt : Inport  Port=60  OutDataTypeStr=uint8
  sTmSigProces_Pw_i16ReqPwrForCool : Inport  Port=61  OutDataTypeStr=int16
  sTmIn_L_s32HvBattCoolFlow1 : Inport  Port=62  OutDataTypeStr=single
  sTmRefriVlvCtrl_X_s32CEXVPosReqAfter3 : Outport  OutDataTypeStr=single
  sTmRefriVlvCtrl_X_s32EEXVPosReqAfter3 : Outport  Port=2  OutDataTypeStr=single
  sTmRefriVlvCtrl_X_s32BEXVPosReqAfter3 : Outport  Port=3  OutDataTypeStr=single
  yTmRefriVlvCtrl_B_HpcCexvMovEnableAfter3 : Outport  Port=4  OutDataTypeStr=boolean
  sTmRefriVlvCtrl_Z_u8CEXVInitStateAfter3 : Outport  Port=5  OutDataTypeStr=uint8
  yTmRefriVlvCtrl_B_CexvCalibReqAfter3 : Outport  Port=6  OutDataTypeStr=boolean
  yTmRefriVlvCtrl_B_HpcEexvMovEnableAfter3 : Outport  Port=7  OutDataTypeStr=boolean
  sTmRefriVlvCtrl_Z_u8EEXVInitStateAfter3 : Outport  Port=8  OutDataTypeStr=uint8
  yTmRefriVlvCtrl_B_EexvCalibReqAfter3 : Outport  Port=9  OutDataTypeStr=boolean
  yTmRefriVlvCtrl_B_HpcBexvMovEnableAfter3 : Outport  Port=10  OutDataTypeStr=boolean
  sTmRefriVlvCtrl_Z_u8BEXVInitStateAfter3 : Outport  Port=11  OutDataTypeStr=uint8
  yTmRefriVlvCtrl_B_BexvCalibReqAfter3 : Outport  Port=12  OutDataTypeStr=boolean
  sTmRefriVlvCtrl_X_s32SM3BexvMaxPosAfter3 : Outport  Port=13  OutDataTypeStr=single
  yTmRefriVlvCtrl_B_EvapBattTLimBexvEnaAfter3 : Outport  Port=14  OutDataTypeStr=boolean
  sTmRefriVlvCtrl_D_u8EexvRefriSwitchStAfter3 : Outport  Port=15  OutDataTypeStr=uint8
  sTmRefriVlvCtrl_D_u8CexvRefriSwitchStAfter3 : Outport  Port=16  OutDataTypeStr=uint8
  sTmRefriVlvCtrl_D_u8BexvRefriSwitchStAfter3 : Outport  Port=17  OutDataTypeStr=uint8
  wires:
  yTmIn_B_CPSRFbSt/1 -> [yTmIn_B_CPSRFbSt]
  sTmIn_D_u8CexvCalibSts/1 -> [sTmIn_D_u8CexvCalibSts]
  ? -> [sTmIn_D_u8EexvCalibSts]
  ? -> [sTmIn_D_u8BexvCalibSts]
  ? -> [sTmDiag_D_u8BexvFltSt]
  sTmDiag_D_u8EexvFltSt/1 -> [sTmDiag_D_u8EexvFltSt]
  sTmDiag_D_u8CexvFltSt/1 -> [sTmDiag_D_u8CexvFltSt]
  ? -> [sTmRefriModeMgr_D_u8HpModeCmd]
  ? -> [sTmSigProces_Te_s32TempInlet]
  ? -> [sTmSigProces_Te_s32CurOutSC]
  ? -> [yTmRefriModeMgr_B_CoolModeInCycle]
  ? -> [sTmSigProces_Te_s32HvBattCooltTFilter]
  ? -> [sTmRefriModeMgr_D_u8HPCurMode]
  ? -> [sTmRefriModeMgr_D_u8HpModeMainState]
  ? -> [sTmSigProces_Te_s32CurSCCalValue]
  yTmRefriModeMgr_B_InterChillDeicing/1 -> [yTmRefriModeMgr_B_InterChillDeicing]
  ? -> [sTmSigProces_Te_s32HvBattCooltTOutFilter]
  ? -> [sTmSigProces_Te_s32TAmb]
  ? -> [sTmSigProces_D_u8CarChrgMode]
  ? -> [sTmIn_D_u8HvBattCoolgReq]
  ? -> [sTmIn_Te_s32HvBattCooltTReq]
  sTmSigProces_Te_s32HeatSH/1 -> [sTmSigProces_Te_s32HeatSH]
  yTmRefriModeMgr_B_CoolOCRMode/1 -> [yTmRefriModeMgr_B_CoolOCRMode]
  sTmSigProces_Te_s32EvapFanReqRamp/1 -> [sTmSigProces_Te_s32EvapFanReqRamp]
  sTmIn_v_s32VehSpdLgt/1 -> [sTmIn_v_s32VehSpdLgt]
  sTmSigProces_Te_s32BattHvMaxFilter/1 -> [sTmSigProces_Te_s32BattHvMaxFilter]
  sTmSigProces_Te_s32EvapFanFilter/1 -> [sTmSigProces_Te_s32EvapFanFilter]
  sTmComprCtrl_n_u16CompRpmReq/1 -> [sTmComprCtrl_n_u16CompRpmReq]
  sTmComprCtrl_n_u16CompMaxRpm/1 -> [sTmComprCtrl_n_u16CompMaxRpm]
  sTmSigProces_Te_s32HeatrAirTReqRamp/1 -> [sTmSigProces_Te_s32HeatrAirTReqRamp]
  sTmSigProces_md_u16BlwHeat/1 -> [sTmSigProces_md_u16BlwHeat]
  sTmSigProces_p_u16PHighSide/1 -> [sTmSigProces_p_u16PHighSide]
  sTmSigProces_Te_s32CompDischarge/1 -> [sTmSigProces_Te_s32CompDischarge]
  yTmIn_B_HmiMaxACReq/1 -> [yTmIn_B_HmiMaxACReq]
  sTmSigProces_Te_s32InletCal/1 -> [sTmSigProces_Te_s32InletCal]
  sTmSigProces_Te_s32CoolSH/1 -> [sTmSigProces_Te_s32CoolSH]
  sTmSigProces_p_u16PLowSide/1 -> [sTmSigProces_p_u16PLowSide]
  sTmSigProces_md_u16BlwCool/1 -> [sTmSigProces_md_u16BlwCool]
  sTmSigProces_Te_s32CurInterSC/1 -> [sTmSigProces_Te_s32CurInterSC]
  yTmHvchCtrl_B_HpcPtcEnad/1 -> [yTmHvchCtrl_B_HpcPtcEnad]
  sTmRefriModeMgr_D_u8HpReqPTCState/1 -> [sTmRefriModeMgr_D_u8HpReqPTCState]
  yTmComprCtrl_B_CompOnReq/1 -> [yTmComprCtrl_B_CompOnReq]
  sTmIn_D_u8HeatPump/1 -> [sTmIn_D_u8HeatPump]
  sTmSigProces_Te_s32HvacHexAirTFilter/1 -> [sTmSigProces_Te_s32HvacHexAirTFilter]
  sTmDiag_D_u8EexvPosnReq2FEnaState/1 -> [sTmDiag_D_u8EexvPosnReq2FEnaState]
  sTmDiag_X_s32EexvPosnReq2F/1 -> [sTmDiag_X_s32EexvPosnReq2F]
  sTmDiag_D_u8EexvMoveEna2FEnaState/1 -> [sTmDiag_D_u8EexvMoveEna2FEnaState]
  yTmDiag_B_EexvMoveEnReq2F/1 -> [yTmDiag_B_EexvMoveEnReq2F]
  sTmDiag_D_u8EexvCal2FEnaState/1 -> [sTmDiag_D_u8EexvCal2FEnaState]
  yTmDiag_B_EexvCalReq2F/1 -> [yTmDiag_B_EexvCalReq2F]
  sTmDiag_D_u8BexvPosnReq2FEnaState/1 -> [sTmDiag_D_u8BexvPosnReq2FEnaState]
  sTmDiag_X_s32BexvPosnReq2F/1 -> [sTmDiag_X_s32BexvPosnReq2F]
  sTmDiag_D_u8BexvMoveEna2FEnaState/1 -> [sTmDiag_D_u8BexvMoveEna2FEnaState]
  yTmDiag_B_BexvMoveEnReq2F/1 -> [yTmDiag_B_BexvMoveEnReq2F]
  sTmDiag_D_u8BexvCal2FEnaState/1 -> [sTmDiag_D_u8BexvCal2FEnaState]
  yTmDiag_B_BexvCalReq2F/1 -> [yTmDiag_B_BexvCalReq2F]
  sTmDiag_D_u8CexvPosnReq2FEnaState/1 -> [sTmDiag_D_u8CexvPosnReq2FEnaState]
  sTmDiag_X_s32CexvPosnReq2F/1 -> [sTmDiag_X_s32CexvPosnReq2F]
  sTmDiag_D_u8CexvMoveEna2FEnaState/1 -> [sTmDiag_D_u8CexvMoveEna2FEnaState]
  yTmDiag_B_CexvMoveEnReq2F/1 -> [yTmDiag_B_CexvMoveEnReq2F]
  sTmDiag_D_u8CexvCal2FEnaState/1 -> [sTmDiag_D_u8CexvCal2FEnaState]
  yTmDiag_B_CexvCalReq2F/1 -> [yTmDiag_B_CexvCalReq2F]
  sTmSigProces_D_u8LargerCoolingFlag/1 -> [sTmSigProces_D_u8LargerCoolingFlag]
  sTmComprCtrl_D_u8HvacFlowLevel/1 -> [sTmComprCtrl_D_u8HvacFlowLevel]
  sTmRefriModeMgr_D_u8ModeSwitchType/1 -> [sTmRefriModeMgr_D_u8ModeSwitchType]
  sTmComprCtrl_D_u8CmprRefriSwitchSt/1 -> [sTmComprCtrl_D_u8CmprRefriSwitchSt]
  sTmIn_X_s32EexvPosSts/1 -> [sTmIn_X_s32EexvPosSts]
  sTmIn_X_s32CexvPosSts/1 -> [sTmIn_X_s32CexvPosSts]
  sTmIn_X_s32BexvPosSts/1 -> [sTmIn_X_s32BexvPosSts]
  sTmSovCtrl_D_u8SOV2RefriSwitchSt/1 -> [sTmSovCtrl_D_u8SOV2RefriSwitchSt]
  sTmDiag_D_u8EvapOutTFltSt/1 -> [sTmDiag_D_u8EvapOutTFltSt]
  sTmDiag_D_u8ChillerOutTFltSt/1 -> [sTmDiag_D_u8ChillerOutTFltSt]
  sTmDiag_D_u8LoSidePFltSt/1 -> [sTmDiag_D_u8LoSidePFltSt]
  sTmDiag_D_u8HiSidePFltSt/1 -> [sTmDiag_D_u8HiSidePFltSt]
  sTmDiag_D_u8OutrCondOutTFltSt/1 -> [sTmDiag_D_u8OutrCondOutTFltSt]
  sTmDiag_D_u8InrCondOutTFltSt/1 -> [sTmDiag_D_u8InrCondOutTFltSt]
  sTmSigProces_Pw_i16ReqPwrForCool/1 -> [sTmSigProces_Pw_i16ReqPwrForCool]
  sTmIn_L_s32HvBattCoolFlow1/1 -> [sTmIn_L_s32HvBattCoolFlow1]
  [sTmRefriVlvCtrl_X_s32CEXVPosReq] -> sTmRefriVlvCtrl_X_s32CEXVPosReqAfter3/1
  [sTmRefriVlvCtrl_X_s32EEXVPosReq] -> sTmRefriVlvCtrl_X_s32EEXVPosReqAfter3/1
  [sTmRefriVlvCtrl_X_s32BEXVPosReq] -> sTmRefriVlvCtrl_X_s32BEXVPosReqAfter3/1
  [yTmRefriVlvCtrl_B_HpcCexvMovEnable] -> yTmRefriVlvCtrl_B_HpcCexvMovEnableAfter3/1
  [sTmRefriVlvCtrl_Z_u8CEXVInitState] -> sTmRefriVlvCtrl_Z_u8CEXVInitStateAfter3/1
  [yTmRefriVlvCtrl_B_CexvCalibReq] -> yTmRefriVlvCtrl_B_CexvCalibReqAfter3/1
  [yTmRefriVlvCtrl_B_HpcEexvMovEnable] -> yTmRefriVlvCtrl_B_HpcEexvMovEnableAfter3/1
  [sTmRefriVlvCtrl_Z_u8EEXVInitState] -> sTmRefriVlvCtrl_Z_u8EEXVInitStateAfter3/1
  [yTmRefriVlvCtrl_B_EexvCalibReq] -> yTmRefriVlvCtrl_B_EexvCalibReqAfter3/1
  [yTmRefriVlvCtrl_B_HpcBexvMovEnable] -> yTmRefriVlvCtrl_B_HpcBexvMovEnableAfter3/1
  [sTmRefriVlvCtrl_Z_u8BEXVInitState] -> sTmRefriVlvCtrl_Z_u8BEXVInitStateAfter3/1
  [yTmRefriVlvCtrl_B_BexvCalibReq] -> yTmRefriVlvCtrl_B_BexvCalibReqAfter3/1
  [sTmRefriVlvCtrl_X_s32SM3BexvMaxPos] -> sTmRefriVlvCtrl_X_s32SM3BexvMaxPosAfter3/1
  [yTmRefriVlvCtrl_B_EvapBattTLimBexvEna] -> yTmRefriVlvCtrl_B_EvapBattTLimBexvEnaAfter3/1
  [sTmRefriVlvCtrl_D_u8EexvRefriSwitchSt] -> sTmRefriVlvCtrl_D_u8EexvRefriSwitchStAfter3/1
  [sTmRefriVlvCtrl_D_u8CexvRefriSwitchSt] -> sTmRefriVlvCtrl_D_u8CexvRefriSwitchStAfter3/1
  [sTmRefriVlvCtrl_D_u8BexvRefriSwitchSt] -> sTmRefriVlvCtrl_D_u8BexvRefriSwitchStAfter3/1

== system ScriptDemo/Create/createPorts/createPortsGotoUpdate/After ==
  note: createPortsGotoUpdate()
      |
      | % 在此路径下执行
      | % 保持原有的信号名
  sTmIn_Pw_s32HvCoolgAllwd : Inport  OutDataTypeStr=single
  xTmComprCtrl_B_CompOnReqCompOn : Inport  Port=2  OutDataTypeStr=boolean
  AllowedPower : Subsystem
  sTmComprCtrl_Pw_s32ElacCmprMaxState : Outport  OutDataTypeStr=single
  yTmComprCtrl_B_HpcCoolgLimd : Outport  Port=2  OutDataTypeStr=boolean
  wires:
  [xTmComprCtrl_B_CompOnReqCompOn] -> AllowedPower/2(xTmComprCtrl_B_CompOnReqCompOn)
  [sTmIn_Pw_s32HvCoolgAllwd] -> AllowedPower/1(sTmIn_Pw_s32HvCoolgAllwd)
  AllowedPower/2(yTmComprCtrl_B_HpcCoolgLimd) -> [yTmComprCtrl_B_HpcCoolgLimd]
  AllowedPower/1(sTmComprCtrl_Pw_s32ElacCmprMaxState) -> [sTmComprCtrl_Pw_s32ElacCmprMaxState]
  sTmIn_Pw_s32HvCoolgAllwd/1 -> [sTmIn_Pw_s32HvCoolgAllwd]
  xTmComprCtrl_B_CompOnReqCompOn/1 -> [xTmComprCtrl_B_CompOnReqCompOn]
  [sTmComprCtrl_Pw_s32ElacCmprMaxState] -> sTmComprCtrl_Pw_s32ElacCmprMaxState/1
  [yTmComprCtrl_B_HpcCoolgLimd] -> yTmComprCtrl_B_HpcCoolgLimd/1

== system ScriptDemo/Create/createPorts/createPortsGotoUpdate/After1 ==
  note: createPortsGotoUpdate( 'mode' , 'pre' )
      |
      | % 在此路径下执行
      | % 使用当前子模型名称作为前缀
  sTmIn_Pw_s32HvCoolgAllwd : Inport  OutDataTypeStr=single
  xTmComprCtrl_B_CompOnReqCompOn : Inport  Port=2  OutDataTypeStr=boolean
  AllowedPower : Subsystem
  rAfter1_Pw_s32ElacCmprMaxState : Outport  OutDataTypeStr=single
  xAfter1_B_HpcCoolgLimd : Outport  Port=2  OutDataTypeStr=boolean
  wires:
  AllowedPower/1(sTmComprCtrl_Pw_s32ElacCmprMaxState) -> [sTmComprCtrl_Pw_s32ElacCmprMaxState]
  [xTmComprCtrl_B_CompOnReqCompOn] -> AllowedPower/2(xTmComprCtrl_B_CompOnReqCompOn)
  [sTmIn_Pw_s32HvCoolgAllwd] -> AllowedPower/1(sTmIn_Pw_s32HvCoolgAllwd)
  AllowedPower/2(yTmComprCtrl_B_HpcCoolgLimd) -> [yTmComprCtrl_B_HpcCoolgLimd]
  sTmIn_Pw_s32HvCoolgAllwd/1 -> [sTmIn_Pw_s32HvCoolgAllwd]
  xTmComprCtrl_B_CompOnReqCompOn/1 -> [xTmComprCtrl_B_CompOnReqCompOn]
  [sTmComprCtrl_Pw_s32ElacCmprMaxState] -> rAfter1_Pw_s32ElacCmprMaxState/1
  [yTmComprCtrl_B_HpcCoolgLimd] -> xAfter1_B_HpcCoolgLimd/1

== system ScriptDemo/Create/createPorts/createPortsGotoUpdate/Before ==
  AllowedPower : Subsystem
  wires:
  [xTmComprCtrl_B_CompOnReqCompOn] -> AllowedPower/2(xTmComprCtrl_B_CompOnReqCompOn)
  [sTmIn_Pw_s32HvCoolgAllwd] -> AllowedPower/1(sTmIn_Pw_s32HvCoolgAllwd)
  AllowedPower/2(yTmComprCtrl_B_HpcCoolgLimd) -> [yTmComprCtrl_B_HpcCoolgLimd]
  AllowedPower/1(sTmComprCtrl_Pw_s32ElacCmprMaxState) -> [sTmComprCtrl_Pw_s32ElacCmprMaxState]

== system ScriptDemo/Create/createPorts/createPortsGotoUpdateLoop/After ==
  sTmIn_Pw_s32HvCoolgAllwd : Inport  OutDataTypeStr=single  OutputFunctionCall=on
  xTmComprCtrl_B_CompOnReqCompOn : Inport  Port=2  OutDataTypeStr=boolean
  xTmComprCtrl_B_AddedSignal : Inport  Port=3  OutDataTypeStr=boolean
  Level3 : Subsystem
  sTmComprCtrl_Pw_s32ElacCmprMaxState : Outport  OutDataTypeStr=single
  yTmComprCtrl_B_HpcCoolgLimd : Outport  Port=2  OutDataTypeStr=boolean
  wires:
  sTmIn_Pw_s32HvCoolgAllwd/1 -> Level3/1(sTmIn_Pw_s32HvCoolgAllwd)  "sTmIn_Pw_s32HvCoolgAllwd"
  xTmComprCtrl_B_CompOnReqCompOn/1 -> Level3/2(xTmComprCtrl_B_CompOnReqCompOn)  "xTmComprCtrl_B_CompOnReqCompOn"
  Level3/1(sTmComprCtrl_Pw_s32ElacCmprMaxState) -> sTmComprCtrl_Pw_s32ElacCmprMaxState/1  "sTmComprCtrl_Pw_s32ElacCmprMaxState"
  Level3/2(yTmComprCtrl_B_HpcCoolgLimd) -> yTmComprCtrl_B_HpcCoolgLimd/1  "yTmComprCtrl_B_HpcCoolgLimd"
  xTmComprCtrl_B_AddedSignal/1 -> Level3/3(xTmComprCtrl_B_AddedSignal)  "xTmComprCtrl_B_AddedSignal"

== system ScriptDemo/Create/createPorts/createPortsGotoUpdateLoop/Before ==
  sTmIn_Pw_s32HvCoolgAllwd : Inport  OutDataTypeStr=single  OutputFunctionCall=on
  xTmComprCtrl_B_CompOnReqCompOn : Inport  Port=2  OutDataTypeStr=boolean
  Level3 : Subsystem
  sTmComprCtrl_Pw_s32ElacCmprMaxState : Outport  OutDataTypeStr=single
  yTmComprCtrl_B_HpcCoolgLimd : Outport  Port=2  OutDataTypeStr=boolean
  wires:
  sTmIn_Pw_s32HvCoolgAllwd/1 -> Level3/1(sTmIn_Pw_s32HvCoolgAllwd)  "sTmIn_Pw_s32HvCoolgAllwd"
  xTmComprCtrl_B_CompOnReqCompOn/1 -> Level3/2(xTmComprCtrl_B_CompOnReqCompOn)  "xTmComprCtrl_B_CompOnReqCompOn"
  Level3/1(sTmComprCtrl_Pw_s32ElacCmprMaxState) -> sTmComprCtrl_Pw_s32ElacCmprMaxState/1  "sTmComprCtrl_Pw_s32ElacCmprMaxState"
  Level3/2(yTmComprCtrl_B_HpcCoolgLimd) -> yTmComprCtrl_B_HpcCoolgLimd/1  "yTmComprCtrl_B_HpcCoolgLimd"
